simulink model "W1985546_20222145_Control_system"  (R2023b)
settings: Solver=VariableStepAuto  StartTime=0.0  StopTime=1000  RelTol=1e-3
libraries: slpidlib x1, SignalEditorBlockLib x1
settings Model: Creator=Acer  LastModifiedBy=Acer

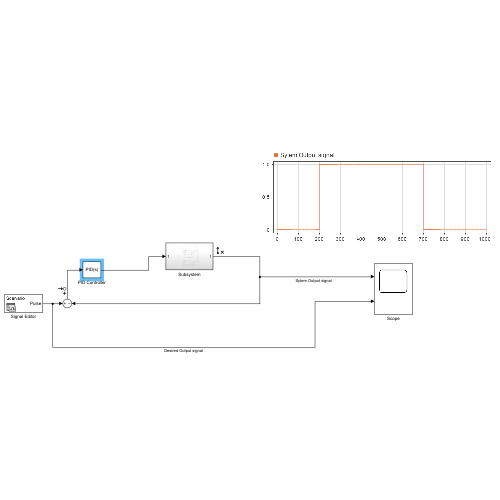
[thumbnail: Simulink's stored preview of the top-level diagram]
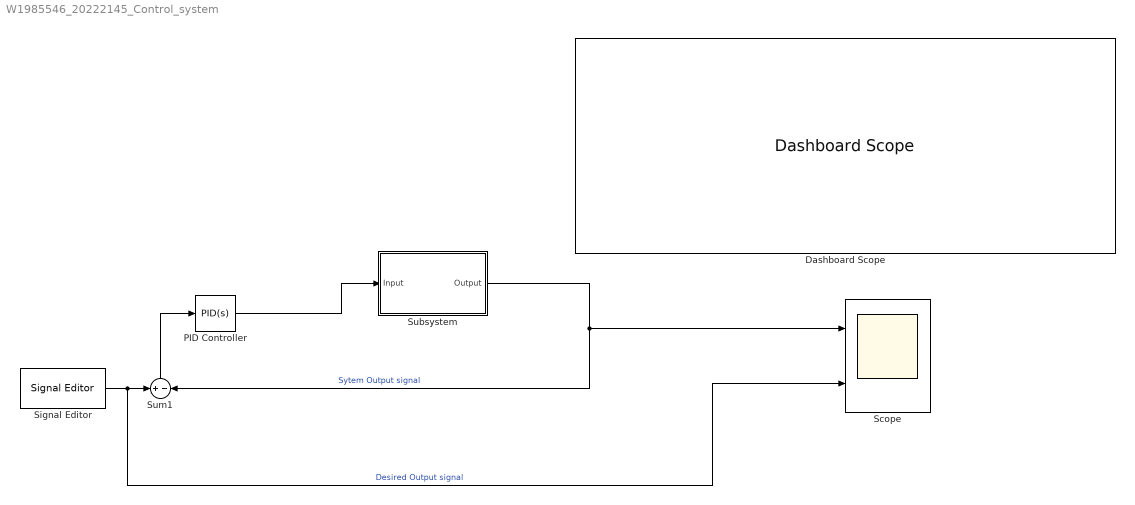
== system W1985546_20222145_Control_system ==
  Dashboard Scope : DashboardScope
  PID Controller : slpidlib/PID Controller  Controller=PID  Form=Parallel  TimeDomain=Continuous-time  UseExternalTs=off  SampleTime=-1  IntegratorMethod=Forward Euler  FilterMethod=Forward Euler  ControllerParametersSource=internal  P=560  I=560  UseKiTs=off  D=250  N=250  UseFilter=on  TunerSelectOption=Frequency Response Based  InitialConditionSource=internal  InitialConditionForIntegrator=0  InitialConditionForFilter=0  DifferentiatorICPrevScaledInput=0  ExternalReset=none  TrackingMode=off  Kt=1  LimitOutput=off  SatLimitsSource=internal  UpperSaturationLimit=inf  LowerSaturationLimit=-inf  LinearizeAsGain=on  AntiWindupMode=none  Kb=1  LimitIntegrator=off  UpperIntegratorSaturationLimit=inf  LowerIntegratorSaturationLimit=-inf  POutMin=[]  POutMax=[]  IOutMin=[]  IOutMax=[]  DOutMin=[]  DOutMax=[]  NOutMin=[]  NOutMax=[]  SumOutMin=[]  SumOutMax=[]  SaturationOutMin=[]  SaturationOutMax=[]  PParamMin=[]  PParamMax=[]  IParamMin=[]  IParamMax=[]  DParamMin=[]  DParamMax=[]  NParamMin=[]  NParamMax=[]  KbParamMin=[]  KbParamMax=[]  KtParamMin=[]  KtParamMax=[]  KbOutMin=[]  KbOutMax=[]  KtOutMin=[]  KtOutMax=[]  IntegratorOutMin=[]  IntegratorOutMax=[]  FilterOutMin=[]  FilterOutMax=[]  SumI1OutMin=[]  SumI1OutMax=[]  SumI2OutMin=[]  SumI2OutMax=[]  SumI3OutMin=[]  SumI3OutMax=[]  SumI4OutMin=[]  SumI4OutMax=[]  SumDOutMin=[]  SumDOutMax=[]  DifferentiatorOutMin=[]  DifferentiatorOutMax=[]  FilterDiffOutCoefMin=[]  FilterDiffOutCoefMax=[]  ReciprocalOutMin=[]  ReciprocalOutMax=[]  SumDenOutMin=[]  SumDenOutMax=[]  SumNumOutMin=[]  SumNumOutMax=[]  DivideOutMin=[]  DivideOutMax=[]  UdiffTsProdOutMin=[]  UdiffTsProdOutMax=[]  NTsProdOutMin=[]  NTsProdOutMax=[]  UintegralTsProdOutMin=[]  UintegralTsProdOutMax=[]  UngainTsProdOutMin=[]  UngainTsProdOutMax=[]  ClampingZeroOutDataTypeStr=Inherit: Inherit via back propagation  ClampingZeroOutMin=[]  ClampingZeroOutMax=[]  FilterDenConstantOutDataTypeStr=Inherit: Inherit via back propagation  FilterDenConstantOutMin=[]  FilterDenConstantOutMax=[]  PCopyOutDataTypeStr=Inherit: Inherit via back propagation  PCopyOutMin=[]  PCopyOutMax=[]  NCopyOutDataTypeStr=Inherit: Inherit via back propagation  NCopyOutMin=[]  NCopyOutMax=[]  IntegratorContinuousStateAttributes=''  IntegratorStateMustResolveToSignalObject=off  IntegratorRTWStateStorageClass=Auto  FilterContinuousStateAttributes=''  FilterStateMustResolveToSignalObject=off  FilterRTWStateStorageClass=Auto  ParallelPVariant=InternalParameters  IdealPVariant=Disabled  IVariant=InternalParameters  DVariant=InternalParameters  IntegratorVariant=Continuous  SatVariant=Disabled  AWVariant=Passthrough  PCopyVariant=Disabled  TRVariant=Disabled  FdbkBlocksVariant=Forward  IdealPFdbkVariant=Disabled  SatFdbkVariant=Disabled  DerivativeFilterVariant=ContFilter  NVariant=InternalParameters  NCopyVariant=Disabled  FilterICVariant=InternalICsFilter  IntegratorICVariant=InternalICs  ExternalResetVariant=Disabled  TRSumVariant=Passthrough  SumFdbkVariant=Disabled  SumVariant=Sum_PID  TsampFilterVariant=InternalTs  TsampNgainVariant=Passthrough  TsampIntegralVariant=Disabled_SignalSpec  ExternalSaturationOutDataTypeStr=Inherit: Same as second input
  Scope : Scope  NumInputPorts=2
  Signal Editor : SignalEditorBlockLib/Signal Editor  FileName=W1985546_20222145_pulse_Speed.mat  ActiveScenario=Scenario  ActiveSignal=Pulse  IsBus=off  OutputBusObjectStr=Bus: BusObject  SampleTime=0  Interpolate=off  ZeroCross=off  OutputAfterFinalValue=Setting to zero  Unit=inherit  PreserveSignalName=on  ApplySigPropsToAllScenarios=on  ApplySigPropsToAllSignals=on
  Subsystem : Subsystem
  Sum1 : Sum  Inputs=+-
  wires:
  Sum1/1 -> PID Controller/1
  Subsystem/1(Output) -> Sum1/2, Scope/1  "Sytem Output signal"
  PID Controller/1 -> Subsystem/1(Input)
  Signal Editor/1 -> Scope/2, Sum1/1  "Desired Output signal"

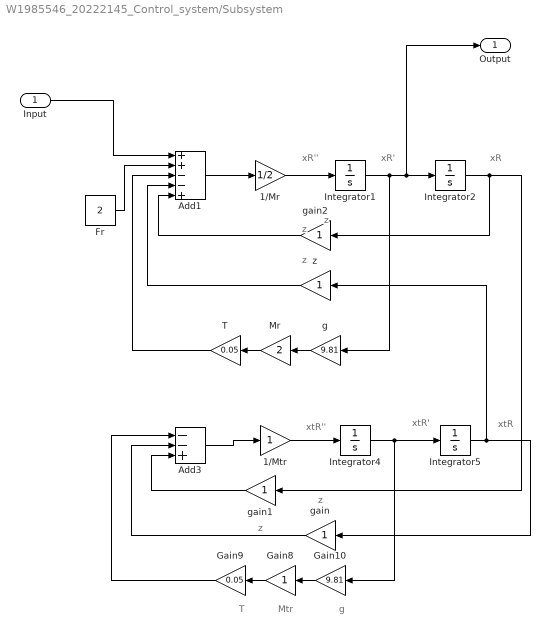
== system W1985546_20222145_Control_system/Subsystem ==
  note: xtR''
  note: xtR
  note: xR
  note: g
  note: xR''
  note: Mtr
  note: xtR'
  note: xR'
  note: T
  note: z
  note: z
  note: z
  note: z
  note: z
  Input : Inport
  1/Mr : Gain  Gain=1/2
  1/Mtr : Gain
  Add1 : Sum  Inputs=++--+
  Add3 : Sum  Inputs=--+
  Fr : Constant  Value=2
  Gain10 : Gain  Gain=9.81
  Gain8 : Gain
  Gain9 : Gain  Gain=0.05
  Integrator{1..2,4..5} (4 alike) : Integrator
  Mr : Gain  Gain=2
  T : Gain  Gain=0.05
  g : Gain  Gain=9.81
  gain : Gain
  gain1 : Gain
  gain2 : Gain
  z : Gain
  Output : Outport
  wires:
  Add1/1 -> 1/Mr/1
  Integrator4/1 -> Integrator5/1, Gain10/1
  Gain8/1 -> Gain9/1
  Add3/1 -> 1/Mtr/1
  Integrator2/1 -> gain1/1, gain2/1
  T/1 -> Add1/3
  Gain10/1 -> Gain8/1
  gain/1 -> Add3/2
  Mr/1 -> T/1
  gain1/1 -> Add3/3
  Gain9/1 -> Add3/1
  z/1 -> Add1/4
  gain2/1 -> Add1/5
  g/1 -> Mr/1
  Input/1 -> Add1/1
  Fr/1 -> Add1/2
  Integrator5/1 -> gain/1, z/1
  Integrator1/1 -> Output/1, Integrator2/1, g/1
  1/Mr/1 -> Integrator1/1
  1/Mtr/1 -> Integrator4/1
